simulink model "TD_YAW_COUPLED"  (R2019b)
settings: Solver=VariableStepAuto  StartTime=0.0  StopTime=10.0  RelTol=1e-3
undefined symbols (not defined in the file): Dt, F_limit_yaw, Jy, k_py, k_yaw
settings Model: Creator=lbend  LastModifiedBy=lbend

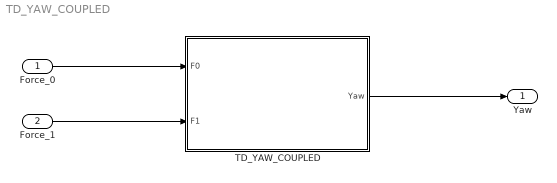
== system TD_YAW_COUPLED ==
  Force_0 : Inport
  "Force_1 " : Inport  Port=2
  TD_YAW_COUPLED : Subsystem
  Yaw : Outport
  wires:
  Force_0/1 -> TD_YAW_COUPLED/1(F0)
  "Force_1 "/1 -> TD_YAW_COUPLED/2(F1)
  TD_YAW_COUPLED/1(Yaw) -> Yaw/1

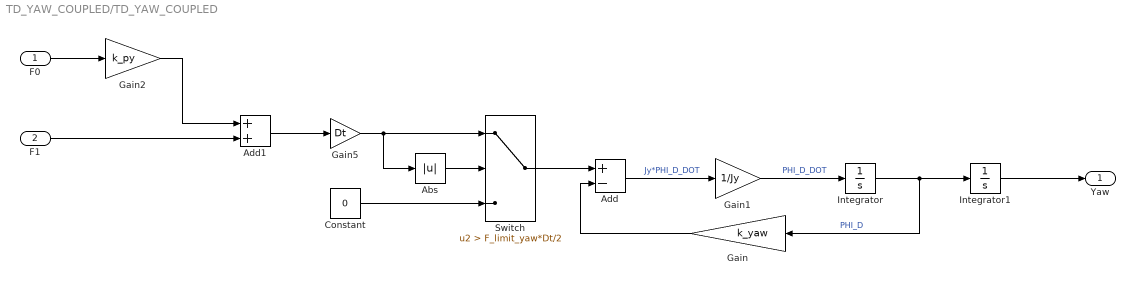
== system TD_YAW_COUPLED/TD_YAW_COUPLED ==
  F0 : Inport
  F1 : Inport  Port=2
  Abs : Abs
  Add : Sum  Inputs=+-
  Add1 : Sum
  Constant : Constant  Value=0
  Gain : Gain  Gain=k_yaw
  Gain1 : Gain  Gain=1/Jy
  Gain2 : Gain  Gain=k_py
  Gain5 : Gain  Gain=Dt
  Integrator : Integrator
  Integrator1 : Integrator
  Switch : Switch  Criteria=u2 > Threshold  Threshold=F_limit_yaw*Dt/2
  Yaw : Outport
  wires:
  Gain2/1 -> Add1/1
  Integrator/1 -> Integrator1/1, Gain/1  "PHI_D"
  Gain/1 -> Add/2
  Add/1 -> Gain1/1  "Jy*PHI_D_DOT"
  Gain1/1 -> Integrator/1  "PHI_D_DOT"
  F1/1 -> Add1/2
  F0/1 -> Gain2/1
  Integrator1/1 -> Yaw/1
  Gain5/1 -> Abs/1, Switch/1
  Constant/1 -> Switch/3
  Add1/1 -> Gain5/1
  Abs/1 -> Switch/2
  Switch/1 -> Add/1
